simulink model "Hydraulic_Actuator"  (R2020a)
settings: Solver=ode4  StartTime=0.0  StopTime=0.25  FixedStep=0.0005  RelTol=1e-3
values from neighbouring files (symbols this model uses):
  Ap = 20.44*10^(-4)    (= 0.002044)    [Parameter.m]
  Beta = 9.81*10^(8)    (= 981000000)    [Parameter.m]
  F = 2.044*10^(3)    (= 2044)    [Parameter.m]
  M = 1000    [Parameter.m]
  P10 = Po    (= 10000000)    [Parameter.m]
  P20 = Po    (= 10000000)    [Parameter.m]
  Vo = 1.063*10^(-4)    (= 0.0001063)    [Parameter.m]
settings Model: Creator=deepa  LastModifiedBy=deepa

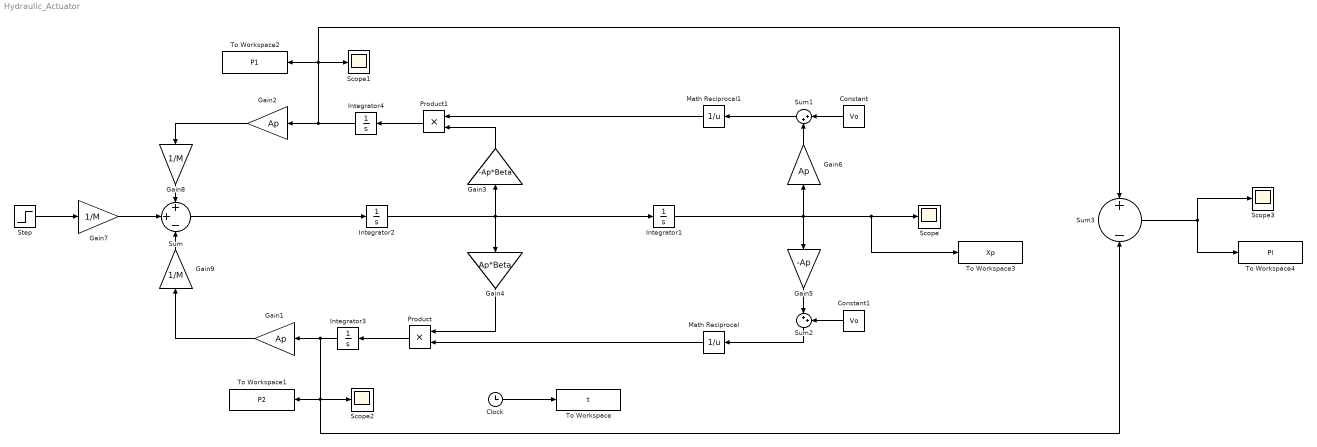
== system Hydraulic_Actuator ==
  Clock : Clock
  Constant : Constant  Value=Vo
  Constant1 : Constant  Value=Vo
  Gain1 : Gain  Gain=Ap
  Gain2 : Gain  Gain=Ap
  Gain3 : Gain  Gain=-Ap*Beta
  Gain4 : Gain  Gain=Ap*Beta
  Gain5 : Gain  Gain=-Ap
  Gain6 : Gain  Gain=Ap
  Gain7 : Gain  Gain=1/M
  Gain8 : Gain  Gain=1/M
  Gain9 : Gain  Gain=1/M
  Integrator1 : Integrator
  Integrator2 : Integrator
  Integrator3 : Integrator  InitialCondition=P20
  Integrator4 : Integrator  InitialCondition=P10
  Math Reciprocal : Math  Operator=reciprocal  SignedPower=on  SaturateOnIntegerOverflow=on
  Math Reciprocal1 : Math  Operator=reciprocal  SignedPower=on  SaturateOnIntegerOverflow=on
  Product : Product
  Product1 : Product
  Scope{,1..3} (4 alike) : Scope
  Step : Step  Time=0  After=F  SampleTime=0
  Sum : Sum  Inputs=++-
  Sum1 : Sum  Inputs=|++
  Sum2 : Sum  Inputs=|++
  Sum3 : Sum  Inputs=+-
  To Workspace : ToWorkspace  VariableName=t  SampleTime=-1
  To Workspace1 : ToWorkspace  VariableName=P2  SampleTime=-1
  To Workspace2 : ToWorkspace  VariableName=P1  SampleTime=-1
  To Workspace3 : ToWorkspace  VariableName=Xp  SampleTime=-1
  To Workspace4 : ToWorkspace  VariableName=Pl  SampleTime=-1
  wires:
  Step/1 -> Gain7/1
  Sum/1 -> Integrator2/1
  Product/1 -> Integrator3/1
  Gain7/1 -> Sum/2
  Gain8/1 -> Sum/1
  Gain9/1 -> Sum/3
  Integrator1/1 -> To Workspace3/1, Scope/1, Gain5/1, Gain6/1
  Constant/1 -> Sum1/1
  Gain6/1 -> Sum1/2
  Gain5/1 -> Sum2/1
  Constant1/1 -> Sum2/2
  Sum2/1 -> Math Reciprocal/1
  Sum1/1 -> Math Reciprocal1/1
  Integrator2/1 -> Integrator1/1, Gain3/1, Gain4/1
  Math Reciprocal1/1 -> Product1/1
  Gain3/1 -> Product1/2
  Product1/1 -> Integrator4/1
  Math Reciprocal/1 -> Product/2
  Gain4/1 -> Product/1
  Clock/1 -> To Workspace/1
  Gain2/1 -> Gain8/1
  Gain1/1 -> Gain9/1
  Integrator3/1 -> To Workspace1/1, Sum3/2, Scope2/1, Gain1/1
  Integrator4/1 -> To Workspace2/1, Sum3/1, Scope1/1, Gain2/1
  Sum3/1 -> To Workspace4/1, Scope3/1
